simulink model "switched_simstate"  (R2020a)
settings: Solver=VariableStepAuto  StartTime=42  StopTime=50  RelTol=1e-3
values from neighbouring files (symbols this model uses):
  dt = 0.001    [param_init.m]    (also in sim_switched.m = options.dt)
undefined symbols (not defined in the file or in its folder): den, num
libraries: simulink x1
settings Model: Creator=kekatos  LastModifiedBy=kekatos
settings DataIOCC: FinalStateName=SimState  InitialState=SimState_previous  LoadInitialState=on  SaveFinalState=on  DSMLogging=off  ReturnWorkspaceOutputs=off

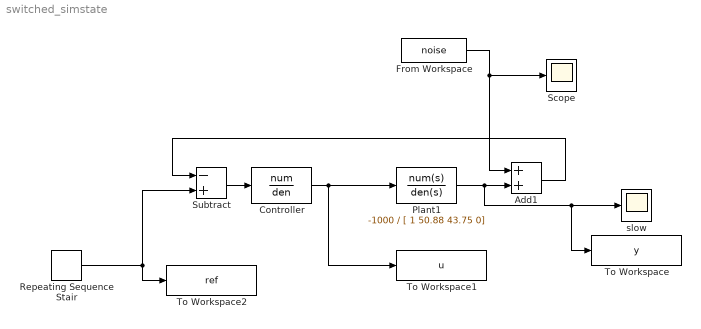
== system switched_simstate ==
  Add1 : Sum
  Controller : TransferFcn  Numerator=num  Denominator=den
  From Workspace : FromWorkspace  VariableName=noise
  Plant1 : TransferFcn  Numerator=-1000  Denominator=[ 1 50.88 43.75 0]
  Repeating Sequence Stair : simulink/Sources/Repeating Sequence Stair  OutValues=[1 1 1 1 1 0 0 0 0 0].'  tsamp=2  OutMin=[]  OutMax=[]  OutDataTypeStr=double  OutputDataTypeScalingMode=double  OutDataType=fixdt(0,8)  ConRadixGroup=Best Precision: Vector-wise  OutScaling=2^-12
  Scope : Scope
  Subtract : Sum  Inputs=-+
  To Workspace : ToWorkspace  VariableName=y  SaveFormat=Structure With Time  SampleTime=dt
  To Workspace1 : ToWorkspace  VariableName=u  SaveFormat=Structure With Time  SampleTime=dt
  To Workspace2 : ToWorkspace  VariableName=ref  SaveFormat=Structure With Time  SampleTime=dt
  slow : Scope
  wires:
  Plant1/1 -> To Workspace/1, slow/1, Add1/2
  Repeating Sequence Stair/1 -> To Workspace2/1, Subtract/2
  Add1/1 -> Subtract/1
  From Workspace/1 -> Scope/1, Add1/1
  Subtract/1 -> Controller/1
  Controller/1 -> Plant1/1, To Workspace1/1
